simulink model "NoSuspensionFrontSSC"  (R2026b)
settings: Solver=VariableStepAuto
settings Model: ModifiedByFormat=The MathWorks, Inc.  Creator=The MathWorks, Inc.  LastModifiedBy=The MathWorks, Inc.
settings DebuggingCC: SubsystemReferenceDiagnosticForUnitTest=warning

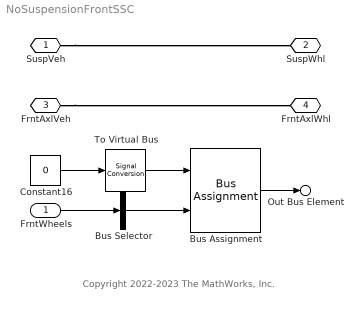
== system NoSuspensionFrontSSC ==
  note: Copyright 2022-2023 The MathWorks, Inc.
  FrntWheels : Inport
  Bus Assignment : BusAssignment  AssignedSignals=FrntSuspWheel.Wheels
  Bus Selector : BusSelector  OutputSignals=Wheels  OutputAsBus=on
  Constant16 : Constant  Value=0  OutDataTypeStr=Bus: FrntSuspBUS  SampleTime=Inf
  To Virtual Bus : SignalConversion  ConversionOutput=Virtual bus  OverrideOpt=off
  SuspVeh : PMIOPort  Side=Left
  SuspWhl : PMIOPort  Port=2  Side=Right
  FrntAxlVeh : PMIOPort  Port=3  Side=Left
  FrntAxlWhl : PMIOPort  Port=4  Side=Right
  Out Bus Element : Outport  PortName=FrntSusp
  wires:
  FrntWheels/1 -> Bus Selector/1
  Constant16/1 -> To Virtual Bus/1
  Bus Assignment/1 -> Out Bus Element/1
  To Virtual Bus/1 -> Bus Assignment/1
  Bus Selector/1 -> Bus Assignment/2
  connections:
  SuspVeh/RConn1 -- SuspWhl/RConn1
  FrntAxlVeh/RConn1 -- FrntAxlWhl/RConn1
